simulink model "yumiao"  (Simulink 9.0)
settings: Solver=FixedStepAuto  StartTime=0.0  StopTime=100  FixedStep=0.01  MaxStep=0.1  RelTol=1e-3  EnableMultiTasking=on
InitFcn:
  | i_sw=17.6
  | pre_x=6
  | t_p=0.3
  | M=1370
  | a=1.1
  | b=1.67
  | C_f=82159
  | C_r=82159
libraries: Solver_SF x1
settings Model: Creator=强哥  LastModifiedBy=yinch
settings DataIOCC: LimitDataPoints=on
settings DebuggingCC: UnderspecifiedInitializationDetection=Simplified  MergeDetectMultiDrivingBlocksExec=error  SolverPrmCheckMsg=warning
settings GRTTargetCC: GeneratePreprocessorConditionals=Disable all
settings ConfigComp: CovHTMLOptions=-sRT=1 -sVT=0 -aTS=1 -bRG=1 -bTC=1 -hTR=0 -nFC=0 -scm=1 -bcm=1 -xEv=0  CovSFcnEnable=off

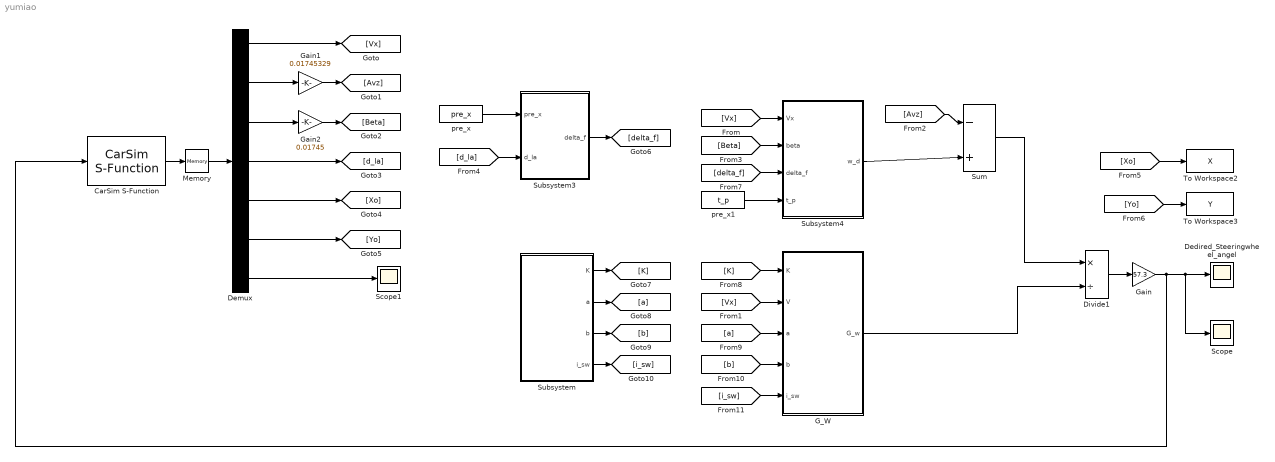
== system yumiao ==
  CarSim S-Function : Solver_SF/CarSim S-Function  Priority=1  VehicleCode=i_i  SIMFILE=simfile
  Dedired_Steeringwheel_angel : Scope
  Demux : Demux  Outputs=7
  Divide1 : Product  Inputs=*/
  G_W : Subsystem
  Gain : Gain  Gain=57.3
  Gain1 : Gain  Gain=0.01745329
  Gain2 : Gain  Gain=0.01745
  Memory : Memory
  Scope : Scope
  Scope1 : Scope
  Subsystem : Subsystem
  Subsystem3 : Subsystem
  Subsystem4 : Subsystem
  Sum : Sum  Inputs=-|+
  To Workspace2 : ToWorkspace  VariableName=X  SampleTime=-1
  To Workspace3 : ToWorkspace  VariableName=Y  SampleTime=-1
  pre_x : Constant  Value=pre_x
  pre_x1 : Constant  Value=t_p
  wires:
  CarSim S-Function/1 -> Memory/1
  Memory/1 -> Demux/1
  Divide1/1 -> Gain/1
  pre_x/1 -> Subsystem3/1(pre_x)
  Demux/3 -> Gain2/1
  Sum/1 -> Divide1/1
  Subsystem4/1(w_d) -> Sum/2
  G_W/1(G_w) -> Divide1/2
  Gain/1 -> Scope/1, Dedired_Steeringwheel_angel/1, CarSim S-Function/1
  Demux/1 -> [Vx]
  [Vx] -> Subsystem4/1(Vx)
  [Vx] -> G_W/2(V)
  Demux/2 -> Gain1/1
  Gain1/1 -> [Avz]
  [Avz] -> Sum/1
  Gain2/1 -> [Beta]
  [Beta] -> Subsystem4/2(beta)
  Demux/4 -> [d_la]
  [d_la] -> Subsystem3/2(d_la)
  Demux/5 -> [Xo]
  Demux/6 -> [Yo]
  [Xo] -> To Workspace2/1
  [Yo] -> To Workspace3/1
  pre_x1/1 -> Subsystem4/4(t_p)
  Subsystem3/1(delta_f) -> [delta_f]
  [delta_f] -> Subsystem4/3(delta_f)
  Subsystem/1(K) -> [K]
  Subsystem/2(a) -> [a]
  Subsystem/3(b) -> [b]
  Subsystem/4("i_sw ") -> [i_sw]
  [K] -> G_W/1(K)
  [a] -> G_W/3(a)
  [b] -> G_W/4(b)
  [i_sw] -> G_W/5(i_sw)
  Demux/7 -> Scope1/1

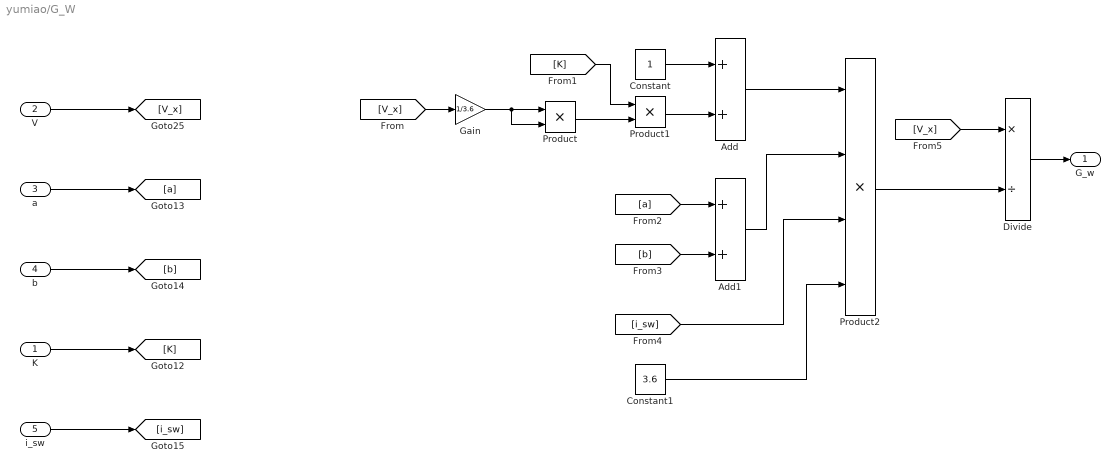
== system yumiao/G_W ==
  K : Inport
  V : Inport  Port=2
  a : Inport  Port=3
  b : Inport  Port=4
  i_sw : Inport  Port=5
  Add : Sum
  Add1 : Sum
  Constant : Constant
  Constant1 : Constant  Value=3.6
  Divide : Product  Inputs=*/
  Gain : Gain  Gain=1/3.6
  Product : Product
  Product1 : Product
  Product2 : Product  Inputs=4
  G_w : Outport
  wires:
  V/1 -> [V_x]
  a/1 -> [a]
  b/1 -> [b]
  K/1 -> [K]
  i_sw/1 -> [i_sw]
  [V_x] -> Gain/1
  Gain/1 -> Product/2, Product/1
  Product/1 -> Product1/2
  [K] -> Product1/1
  Product1/1 -> Add/2
  Constant/1 -> Add/1
  [a] -> Add1/1
  [b] -> Add1/2
  Add/1 -> Product2/1
  Add1/1 -> Product2/2
  [i_sw] -> Product2/3
  Constant1/1 -> Product2/4
  Product2/1 -> Divide/2
  [V_x] -> Divide/1
  Divide/1 -> G_w/1

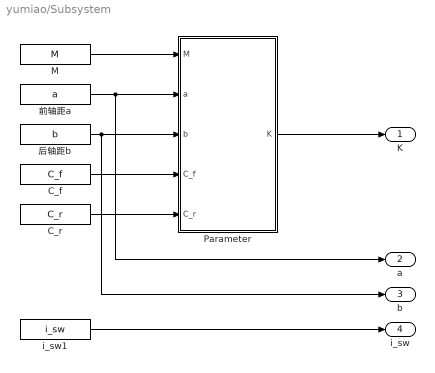
== system yumiao/Subsystem ==
  C_f : Constant  Value=C_f
  C_r : Constant  Value=C_r
  M : Constant  Value=M
  Parameter : Subsystem
  i_sw1 : Constant  Value=i_sw
  前轴距a : Constant  Value=a
  后轴距b : Constant  Value=b
  K : Outport
  a : Outport  Port=2
  b : Outport  Port=3
  "i_sw " : Outport  Port=4
  wires:
  前轴距a/1 -> a/1, Parameter/2(a)
  M/1 -> Parameter/1(M)
  后轴距b/1 -> b/1, Parameter/3(b)
  Parameter/1(K) -> K/1
  C_f/1 -> Parameter/4(C_f)
  C_r/1 -> Parameter/5(C_r)
  i_sw1/1 -> "i_sw "/1

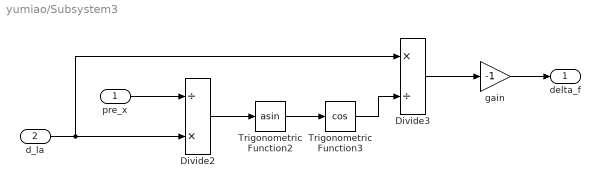
== system yumiao/Subsystem3 ==
  pre_x : Inport
  d_la : Inport  Port=2
  Divide2 : Product  Inputs=/*
  Divide3 : Product  Inputs=*/
  Trigonometric Function2 : Trigonometry  Operator=asin
  Trigonometric Function3 : Trigonometry  Operator=cos
  gain : Gain  Gain=-1
  delta_f : Outport
  wires:
  d_la/1 -> Divide3/1, Divide2/2
  Divide3/1 -> gain/1
  Divide2/1 -> Trigonometric Function2/1
  Trigonometric Function3/1 -> Divide3/2
  Trigonometric Function2/1 -> Trigonometric Function3/1
  pre_x/1 -> Divide2/1
  gain/1 -> delta_f/1

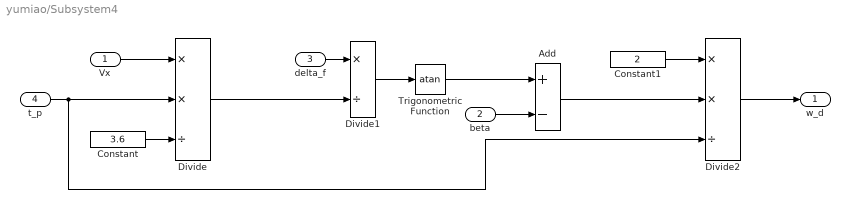
== system yumiao/Subsystem4 ==
  Vx : Inport
  beta : Inport  Port=2
  delta_f : Inport  Port=3
  t_p : Inport  Port=4
  Add : Sum  Inputs=+-
  Constant : Constant  Value=3.6
  Constant1 : Constant  Value=2
  Divide : Product  Inputs=**/
  Divide1 : Product  Inputs=*/
  Divide2 : Product  Inputs=**/
  Trigonometric Function : Trigonometry  Operator=atan
  w_d : Outport
  wires:
  beta/1 -> Add/2
  Vx/1 -> Divide/1
  delta_f/1 -> Divide1/1
  t_p/1 -> Divide/2, Divide2/3
  Constant/1 -> Divide/3
  Divide/1 -> Divide1/2
  Divide1/1 -> Trigonometric Function/1
  Trigonometric Function/1 -> Add/1
  Constant1/1 -> Divide2/1
  Add/1 -> Divide2/2
  Divide2/1 -> w_d/1

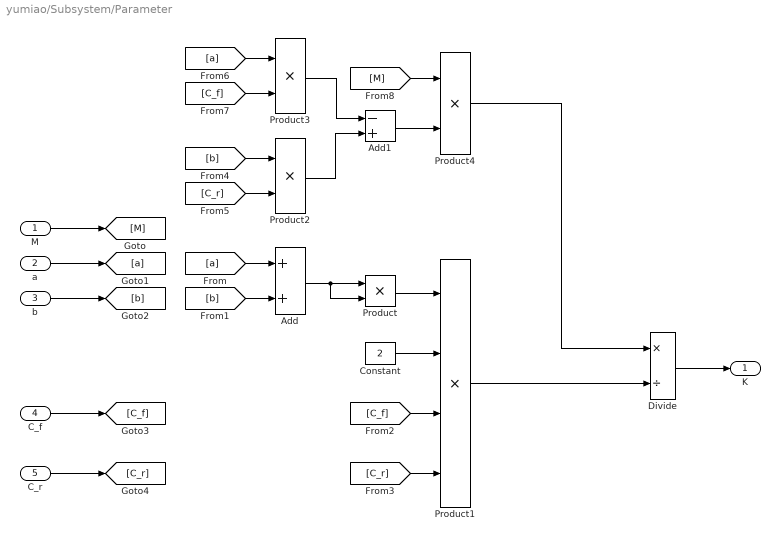
== system yumiao/Subsystem/Parameter ==
  M : Inport
  a : Inport  Port=2
  b : Inport  Port=3
  C_f : Inport  Port=4
  C_r : Inport  Port=5
  Add : Sum
  Add1 : Sum  Inputs=-+
  Constant : Constant  Value=2
  Divide : Product  Inputs=*/
  Product{,2..4} (4 alike) : Product
  Product1 : Product  Inputs=4
  K : Outport
  wires:
  Add/1 -> Product/2, Product/1
  Product/1 -> Product1/1
  Product1/1 -> Divide/2
  M/1 -> [M]
  a/1 -> [a]
  b/1 -> [b]
  C_f/1 -> [C_f]
  C_r/1 -> [C_r]
  [a] -> Add/1
  [b] -> Add/2
  [C_f] -> Product1/3
  [C_r] -> Product1/4
  Constant/1 -> Product1/2
  [b] -> Product2/1
  [C_r] -> Product2/2
  [C_f] -> Product3/2
  [a] -> Product3/1
  Product3/1 -> Add1/1
  Product2/1 -> Add1/2
  Add1/1 -> Product4/2
  [M] -> Product4/1
  Product4/1 -> Divide/1
  Divide/1 -> K/1
